simulink model "m"  (R2016b)
settings: Solver=VariableStepAuto  StartTime=0.0  StopTime=10.0  RelTol=1e-3
settings Model: Creator=ASUS  LastModifiedBy=ASUS

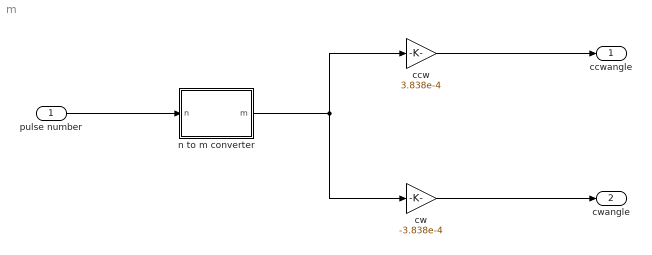
== system m ==
  pulse number : Inport
  ccw : Gain  Gain=3.838e-4
  cw : Gain  Gain=-3.838e-4
  n to m converter : MATLAB Function  TreatAsAtomicUnit=on
  ccwangle : Outport
  cwangle : Outport  Port=2
  wires:
  pulse number/1 -> n to m converter/1(n)
  n to m converter/1(m) -> ccw/1, cw/1
  ccw/1 -> ccwangle/1
  cw/1 -> cwangle/1

== matlab function m/n to m converter ==
  data: n input; m output
function m = fcn(n)
% this function keep our angle between pi and -pi
q = round(n/4096)-1;
m = n - q * 4096;
end
